simulink model "detectorDTMFv_nova"  (R2015a)
settings: Solver=ode45  StartTime=0.0  StopTime=10  RelTol=1e-3
undefined symbols (not defined in the file or in its folder): fa1
undefined symbols (not defined in the file): spf1
libraries: dsparch4 x12, dspvision x2, dspsrcs4 x2
settings Model: Creator=aluno  LastModifiedBy=aluno

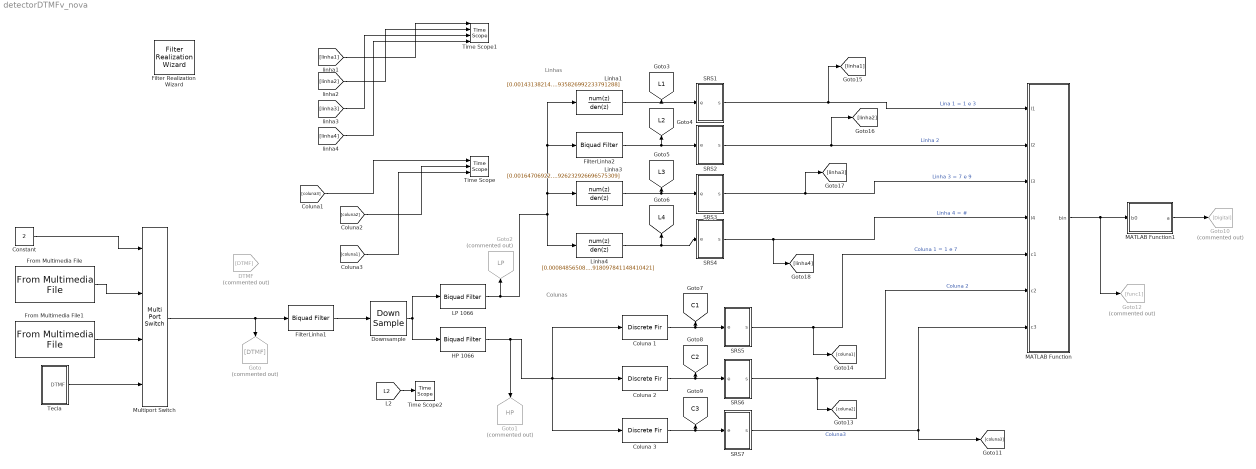
== system detectorDTMFv_nova ==
  note: Colunas
  note: Linhas
  Coluna 1 : DiscreteFir  Tag=BlockMethodSubSystem  Coefficients=[0.0162374776061879368 0.00189985661140890452 -0.00797907219847647162 -0.0052479937717645319 0.00711016072981206747 0.00994959173688526183 -0.004947856232688801 -0.0134569820625869124 -0.000253952320820913235 0.0161841189423569572 0.00648786614938951737 -0.015546033116355204 -0.0142422778845492579 0.0123011904003162455 0.020662915544833009 -0.00502839342402886316 -0.0254317147244396899 -0.00430154976592201765 0.0259053247088500034 0.0154089086154453655 -0.0223513453420253506 -0.0252581254312456739 0.0137329360710826773 0.0327518005541912877 -0.00195023169392464796 -0.0352357630400336602 -0.0120135916294035645 0.0324725455811842589 0.0250613597548236811 -0.0238106275094853714 -0.035341140965640179 0.0109201536347342254 0.0403511098959608225 0.00454288360450943313 -0.0393003808148319617 -0.0196726822859361571 0.0319801461843528603 0.0319801461843528603 -0.0196726822859361571 -0.0393003808148319617 0.00454288360450943313 0.0403511098959608225 0.0109201536347342254 -0.035341140965640179 -0.0238106275094853714 0.0250613597548236811 0.0324725455811842589 -0.0120135916294035645 -0.0352357630400336602 -0.00195023169392464796 0.0327518005541912877 0.0137329360710826773 -0.0252581254312456739 -0.0223513453420253506 0.0154089086154453655 0.0259053247088500034 -0.00430154976592201765 -0.0254317147244396899 -0.00502839342402886316 0.020662915544833009 0.0123011904003162455 -0.0142422778845492579 -0.015546033116355204 0.00648786614938951737 0.0161841189423569572 -0.000253952320820913235 -0.0134569820625869124 -0.004947856232688801 0.00994959173688526183 0.00711016072981206747 -0.0052479937717645319 -0.00797907219847647162 0.00189985661140890452 0.0162374776061879368]  InputProcessing=Columns as channels (frame based)
  Coluna 2 : DiscreteFir  Tag=BlockMethodSubSystem  Coefficients=[0.0151609358216046233 0.00947495343349298927 -0.0146508717306113884 -0.00105872890071495823 0.00918832200093996215 0.00869381341841268633 -0.0152655644424472808 -0.00814107176471721115 0.0147925932332998757 0.0127477000713067754 -0.0175823788993001162 -0.0151052177040993923 0.0180679752451277792 0.0192083709848808286 -0.0191711594948643961 -0.0227113888358491493 0.0191652238273957339 0.0267522427716407989 -0.0189311110191219371 -0.0305289457692412315 0.0179327879619009534 0.0342765820241483776 -0.0164300130975231704 -0.0376548966600824472 0.0143049369115090964 0.0406609187674431688 -0.0117262623087099286 -0.043127450615960447 0.00868997394253513689 0.0449559783178955022 -0.00535632534591356721 -0.046091514358570472 0.00181093739417893286 0.0464677162435992649 0.00181093739417893286 -0.046091514358570472 -0.00535632534591356721 0.0449559783178955022 0.00868997394253513689 -0.043127450615960447 -0.0117262623087099286 0.0406609187674431688 0.0143049369115090964 -0.0376548966600824472 -0.0164300130975231704 0.0342765820241483776 0.0179327879619009534 -0.0305289457692412315 -0.0189311110191219371 0.0267522427716407989 0.0191652238273957339 -0.0227113888358491493 -0.0191711594948643961 0.0192083709848808286 0.0180679752451277792 -0.0151052177040993923 -0.0175823788993001162 0.0127477000713067754 0.0147925932332998757 -0.00814107176471721115 -0.0152655644424472808 0.00869381341841268633 0.00918832200093996215 -0.00105872890071495823 -0.0146508717306113884 0.00947495343349298927 0.0151609358216046233]  InputProcessing=Columns as channels (frame based)
  Coluna 3 : DiscreteFir  Tag=BlockMethodSubSystem  Coefficients=[0.00988513023850831618 -0.0150839385628058591 -0.012276056219741845 0.00793493611486074772 0.00624928738101373886 -0.0154557718125388887 -0.00580602331170108898 0.0194847183612866931 0.00170258274655131253 -0.0239671147608122893 0.00374191930103570658 0.0270475037862077383 -0.0109223335109471052 -0.028320544283840763 0.0191883198599795482 0.0272259567957319551 -0.0278505151864056333 -0.0234560510640422493 0.0360331366276040732 0.0169923009575104825 -0.0428124432863375426 -0.0081801447891480146 0.0473482486516168463 -0.00236615855399630731 -0.0489985066204024072 0.0137299516321145107 0.0473977728496665293 -0.0248925638188108173 -0.0425415916558437579 0.0348110051185492875 0.0348110051185492875 -0.0425415916558437579 -0.0248925638188108173 0.0473977728496665293 0.0137299516321145107 -0.0489985066204024072 -0.00236615855399630731 0.0473482486516168463 -0.0081801447891480146 -0.0428124432863375426 0.0169923009575104825 0.0360331366276040732 -0.0234560510640422493 -0.0278505151864056333 0.0272259567957319551 0.0191883198599795482 -0.028320544283840763 -0.0109223335109471052 0.0270475037862077383 0.00374191930103570658 -0.0239671147608122893 0.00170258274655131253 0.0194847183612866931 -0.00580602331170108898 -0.0154557718125388887 0.00624928738101373886 0.00793493611486074772 -0.012276056219741845 -0.0150839385628058591 0.00988513023850831618]  InputProcessing=Columns as channels (frame based)
  Constant : Constant  Value=2
  DTMF : From  Commented=on  GotoTag=DTMF
  Downsample : DownSample  N=8  RateOptions=Allow multirate processing
  Filter Realization Wizard : dsparch4/Filter Realization Wizard
  FilterLinha1 : dsparch4/Biquad Filter  Tag=BlockMethodSubSystem  IIRFiltStruct=Direct form II  CoeffSource=Specify via dialog  BiQuadCoeffs=[1 2 1 1 -1.77399903150737015 0.912639318363765439;1 2 1 1 -1.76215470273778285 0.79641905117053291]  a0Flag=Warning  IC=0  ICnum=0  ICden=0  InputProcessing=Columns as channels (frame based)  denAccumFracLength=30  denProdOutputFracLength=30  secondMemoryFracLength=15  roundingMode=Floor  overflowMode=off  ScaleValues=[0.0346600717140988085;0.00856608710818747114;0.841395141645195133]  optimizeScaleValues=on  ScaleValueMode=Specify via input port (g)  scaleValueFracLength=14  FilterSource=Specify via dialog  FilterObject=Hm_biquad
  FilterLinha2 : dsparch4/Biquad Filter  Tag=BlockMethodSubSystem  IIRFiltStruct=Direct form II  CoeffSource=Specify via dialog  BiQuadCoeffs=[1 -1.4206643064571538 1 1 -1.25491628037472003 0.985502558796195638;1 -1.1033582980484935 1 1 -1.27745221072506698 0.985676226822505219]  a0Flag=Warning  IC=0  ICnum=0  ICden=0  InputProcessing=Columns as channels (frame based)  denAccumFracLength=30  denProdOutputFracLength=30  secondMemoryFracLength=15  roundingMode=Floor  overflowMode=off  ScaleValues=[0.0998036605233421636;0.0998036605233421636;1]  optimizeScaleValues=on  ScaleValueMode=Specify via input port (g)  scaleValueFracLength=14  FilterSource=Specify via dialog  FilterObject=Hm_biquad
  From Multimedia File : dspvision/From Multimedia File  inputFilename=/home/aluno/Downloads/DTMF.ogg  loop=on  numPlays=inf  outputStreams=Audio only  videoDataType=single  audioDataType=double  inheritSampleTime=on  userDefinedSampleTime=1/30  noAudioOutput=off  isIntensityVideo=off  fourcc=RGB  colorVideoFormat=Separate color signals  outputEOF=off  dataOrg=Column-major  audioFrameSize=spf1  computeAudioFrameSize=off  outSamplingMode=Sample based
  From Multimedia File1 : dspvision/From Multimedia File  inputFilename=/home/aluno/Downloads/7913#.ogg  loop=on  numPlays=inf  outputStreams=Audio only  videoDataType=single  audioDataType=double  inheritSampleTime=on  userDefinedSampleTime=1/30  noAudioOutput=off  isIntensityVideo=off  fourcc=RGB  colorVideoFormat=Separate color signals  outputEOF=off  dataOrg=Column-major  audioFrameSize=spf1  computeAudioFrameSize=off  outSamplingMode=Sample based
  Goto : Goto  Commented=on  GotoTag=DTMF
  Goto1 : Goto  Commented=on  GotoTag=HP  TagVisibility=global
  Goto10 : Goto  Commented=on  GotoTag=Digital
  Goto12 : Goto  Commented=on  GotoTag=func1
  Goto2 : Goto  Commented=on  GotoTag=LP  TagVisibility=global
  HP 1066 : dsparch4/Biquad Filter  Tag=BlockMethodSubSystem  IIRFiltStruct=Direct form II  CoeffSource=Specify via dialog  BiQuadCoeffs=[1 -2 1 1 -0.584098631504043841 0.792871341403187047;1 -2 1 1 0.426036160749820147 0.290070169958779767]  a0Flag=Warning  IC=0  ICnum=0  ICden=0  InputProcessing=Columns as channels (frame based)  denAccumFracLength=30  denProdOutputFracLength=30  secondMemoryFracLength=15  roundingMode=Floor  overflowMode=off  ScaleValues=[0.594242493226807778;0.216008502302239891;0.841395141645195133]  optimizeScaleValues=on  ScaleValueMode=Specify via input port (g)  scaleValueFracLength=14  FilterSource=Specify via dialog  FilterObject=Hm_biquad
  LP 1066 : dsparch4/Biquad Filter  Tag=BlockMethodSubSystem  IIRFiltStruct=Direct form II  CoeffSource=Specify via dialog  BiQuadCoeffs=[1 2 1 1 -0.665333766450005193 0.79613348517815774;1 2 1 1 -1.16290921522145752 0.47295210928305087]  a0Flag=Warning  IC=0  ICnum=0  ICden=0  InputProcessing=Columns as channels (frame based)  denAccumFracLength=30  denProdOutputFracLength=30  secondMemoryFracLength=15  roundingMode=Floor  overflowMode=off  ScaleValues=[0.282699929682038165;0.0775107235153982832;0.841395141645195133]  optimizeScaleValues=on  ScaleValueMode=Specify via input port (g)  scaleValueFracLength=14  FilterSource=Specify via dialog  FilterObject=Hm_biquad
  Linha1 : DiscreteFilter  Tag=BlockMethodSubSystem  Numerator=[0.00143138214148962246 -0.00399928386900759263 0.00421549467129527129 0 -0.00421549467129527129 0.00399928386900759263 -0.00143138214148962246]  Denominator=[1 -4.15803677575891317 8.69712495446401412 -10.7962985508542388 8.50695759347203584 -3.9781853030165335 0.935826992233791288]  InputProcessing=Columns as channels (frame based)  a0EqualsOne=on
  Linha3 : DiscreteFilter  Tag=BlockMethodSubSystem  Numerator=[0.00164706922346999091 -0.00370526492343735631 0.00371166563158928245 0 -0.00371166563158928245 0.00370526492343735631 -0.00164706922346999091]  Denominator=[1 -3.34565745513575852 6.65482815014997531 -7.90884772414054105 6.48700170175998547 -3.17902828471224197 0.926232926696575309]  InputProcessing=Columns as channels (frame based)  a0EqualsOne=on
  Linha4 : DiscreteFilter  Tag=BlockMethodSubSystem  Numerator=[0.000848565081379532146 -0.00160409606198937496 0.00157713327916364325 -6.54306174870359165e-21 -0.00157713327916364325 0.00160409606198937496 -0.000848565081379532146]  Denominator=[1 -2.82691943332089002 5.57865613790708803 -6.33091320195414919 5.42200709739372488 -2.67037232087107812 0.918097841148410421]  InputProcessing=Columns as channels (frame based)  a0EqualsOne=on
  MATLAB Function : MATLAB Function  TreatAsAtomicUnit=on
  MATLAB Function1 : MATLAB Function  TreatAsAtomicUnit=on
  Multiport Switch : MultiPortSwitch
  SRS1 : Subsystem
  SRS2 : Subsystem
  SRS3 : Subsystem
  SRS4 : Subsystem
  SRS5 : Subsystem
  SRS6 : Subsystem
  SRS7 : Subsystem
  Tecla : Subsystem  mask{linha=697, coluna=1209, spf1=spf1, fa1=fa1}
      mask prompts: linha "Frequencia da linha [linha]"; coluna "Frequencia da coluna [coluna]"; spf1 "Amostras por quadro [spf1]"; fa1 "Frequencia de Amostragem [fa1]"
  Time Scope : TimeScope  DefaultConfigurationName=spbscopes.TimeScopeBlockCfg  NumInputPorts=3
  Time Scope1 : TimeScope  DefaultConfigurationName=spbscopes.TimeScopeBlockCfg  NumInputPorts=4
  Time Scope2 : TimeScope  DefaultConfigurationName=spbscopes.TimeScopeBlockCfg
  tag scope: C1=global, C2=global, C3=global, L1=global, L2=global, L3=global, L4=global
  wires:
  Constant/1 -> Multiport Switch/1
  From Multimedia File/1 -> Multiport Switch/2
  From Multimedia File1/1 -> Multiport Switch/3
  Tecla/1(DTMF) -> Multiport Switch/4
  FilterLinha1/1 -> Downsample/1
  Multiport Switch/1 -> FilterLinha1/1, Goto/1
  Downsample/1 -> HP 1066/1, LP 1066/1
  SRS4/1(s) -> [linha4], MATLAB Function/4(l4)  "Linha 4 = #"
  SRS3/1(s) -> [linha3], MATLAB Function/3(l3)  "Linha 3 = 7 e 9"
  SRS2/1(s) -> [linha2], MATLAB Function/2(l2)  "Linha 2"
  SRS1/1(s) -> [linha1], MATLAB Function/1(l1)  "Lina 1 = 1 e 3"
  LP 1066/1 -> Goto2/1, Linha4/1, Linha3/1, FilterLinha2/1, Linha1/1
  SRS7/1(s) -> MATLAB Function/7(c3), [coluna3]  "Coluna3"
  SRS6/1(s) -> [coluna2], MATLAB Function/6(c2)  "Coluna 2"
  SRS5/1(s) -> [coluna1], MATLAB Function/5(c1)  "Coluna 1 = 1 e 7"
  Coluna 2/1 -> SRS6/1(e), [C2]
  Coluna 3/1 -> SRS7/1(e), [C3]
  Coluna 1/1 -> SRS5/1(e), [C1]
  HP 1066/1 -> Goto1/1, Coluna 3/1, Coluna 2/1, Coluna 1/1
  MATLAB Function/1(bin) -> Goto12/1, MATLAB Function1/1(b0)
  MATLAB Function1/1(a) -> Goto10/1
  Linha1/1 -> SRS1/1(e), [L1]
  Linha3/1 -> SRS3/1(e), [L3]
  Linha4/1 -> [L4], SRS4/1(e)
  [coluna3] -> Time Scope/1
  [coluna2] -> Time Scope/2
  [coluna1] -> Time Scope/3
  [linha1] -> Time Scope1/1
  [linha2] -> Time Scope1/2
  [linha3] -> Time Scope1/3
  [linha4] -> Time Scope1/4
  [L2] -> Time Scope2/1
  FilterLinha2/1 -> SRS2/1(e), [L2]

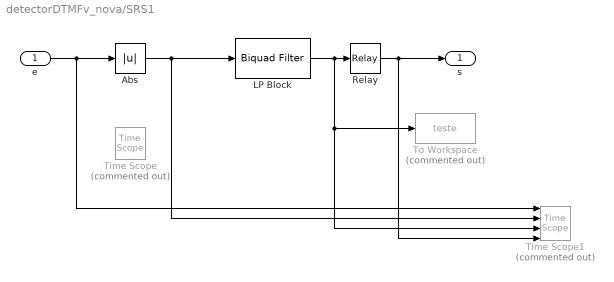
== system detectorDTMFv_nova/SRS1 ==
  e : Inport
  Abs : Abs
  LP Block : dsparch4/Biquad Filter  Tag=BlockMethodSubSystem  IIRFiltStruct=Direct form II  CoeffSource=Specify via dialog  BiQuadCoeffs=[1 2 1 1 -1.9659013837346071 0.967099117650403017]  a0Flag=Warning  IC=0  ICnum=0  ICden=0  InputProcessing=Columns as channels (frame based)  denAccumFracLength=30  denProdOutputFracLength=30  secondMemoryFracLength=15  roundingMode=Floor  overflowMode=off  ScaleValues=[0.000299433478949018132;0.841395141645195133]  optimizeScaleValues=on  ScaleValueMode=Specify via input port (g)  scaleValueFracLength=14  FilterSource=Specify via dialog  FilterObject=Hm_biquad
  Relay : Relay  OnSwitchValue=0.12  OffSwitchValue=0.05  ZeroCross=off
  Time Scope : TimeScope  Commented=on  DefaultConfigurationName=spbscopes.TimeScopeBlockCfg
  Time Scope1 : TimeScope  Commented=on  DefaultConfigurationName=spbscopes.TimeScopeBlockCfg  NumInputPorts=4
  To Workspace : ToWorkspace  Commented=on  VariableName=teste  SaveFormat=Timeseries  SampleTime=-1
  s : Outport
  wires:
  e/1 -> Time Scope1/1, Abs/1
  Abs/1 -> LP Block/1, Time Scope1/2
  Relay/1 -> Time Scope1/4, s/1
  LP Block/1 -> Relay/1, To Workspace/1, Time Scope1/3

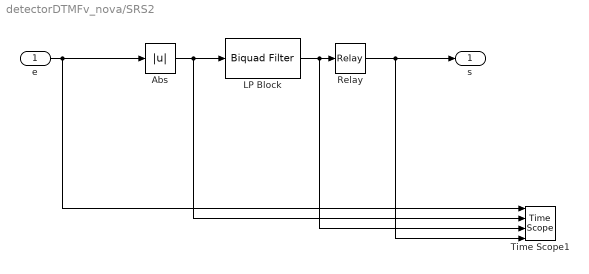
== system detectorDTMFv_nova/SRS2 ==
  e : Inport
  Abs : Abs
  LP Block : dsparch4/Biquad Filter  Tag=BlockMethodSubSystem  IIRFiltStruct=Direct form II  CoeffSource=Specify via dialog  BiQuadCoeffs=[1 2 1 1 -1.9659013837346071 0.967099117650403017]  a0Flag=Warning  IC=0  ICnum=0  ICden=0  InputProcessing=Columns as channels (frame based)  denAccumFracLength=30  denProdOutputFracLength=30  secondMemoryFracLength=15  roundingMode=Floor  overflowMode=off  ScaleValues=[0.000299433478949018132;0.841395141645195133]  optimizeScaleValues=on  ScaleValueMode=Specify via input port (g)  scaleValueFracLength=14  FilterSource=Specify via dialog  FilterObject=Hm_biquad
  Relay : Relay  OnSwitchValue=0.12  OffSwitchValue=0.05  ZeroCross=off
  Time Scope1 : TimeScope  DefaultConfigurationName=spbscopes.TimeScopeBlockCfg  NumInputPorts=4
  s : Outport
  wires:
  e/1 -> Time Scope1/1, Abs/1
  Abs/1 -> LP Block/1, Time Scope1/2
  Relay/1 -> Time Scope1/4, s/1
  LP Block/1 -> Time Scope1/3, Relay/1

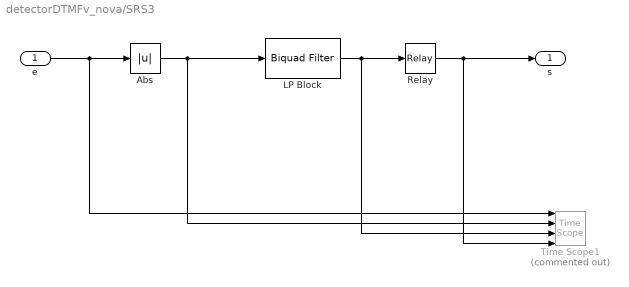
== system detectorDTMFv_nova/SRS3 ==
  e : Inport
  Abs : Abs
  LP Block : dsparch4/Biquad Filter  Tag=BlockMethodSubSystem  IIRFiltStruct=Direct form II  CoeffSource=Specify via dialog  BiQuadCoeffs=[1 2 1 1 -1.9659013837346071 0.967099117650403017]  a0Flag=Warning  IC=0  ICnum=0  ICden=0  InputProcessing=Columns as channels (frame based)  denAccumFracLength=30  denProdOutputFracLength=30  secondMemoryFracLength=15  roundingMode=Floor  overflowMode=off  ScaleValues=[0.000299433478949018132;0.841395141645195133]  optimizeScaleValues=on  ScaleValueMode=Specify via input port (g)  scaleValueFracLength=14  FilterSource=Specify via dialog  FilterObject=Hm_biquad
  Relay : Relay  OnSwitchValue=0.12  OffSwitchValue=0.05  ZeroCross=off
  Time Scope1 : TimeScope  Commented=on  DefaultConfigurationName=spbscopes.TimeScopeBlockCfg  NumInputPorts=4
  s : Outport
  wires:
  LP Block/1 -> Time Scope1/3, Relay/1
  e/1 -> Time Scope1/1, Abs/1
  Abs/1 -> LP Block/1, Time Scope1/2
  Relay/1 -> Time Scope1/4, s/1

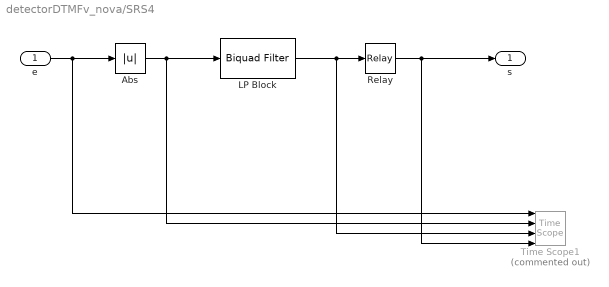
== system detectorDTMFv_nova/SRS4 ==
  e : Inport
  Abs : Abs
  LP Block : dsparch4/Biquad Filter  Tag=BlockMethodSubSystem  IIRFiltStruct=Direct form II  CoeffSource=Specify via dialog  BiQuadCoeffs=[1 2 1 1 -1.9659013837346071 0.967099117650403017]  a0Flag=Warning  IC=0  ICnum=0  ICden=0  InputProcessing=Columns as channels (frame based)  denAccumFracLength=30  denProdOutputFracLength=30  secondMemoryFracLength=15  roundingMode=Floor  overflowMode=off  ScaleValues=[0.000299433478949018132;0.841395141645195133]  optimizeScaleValues=on  ScaleValueMode=Specify via input port (g)  scaleValueFracLength=14  FilterSource=Specify via dialog  FilterObject=Hm_biquad
  Relay : Relay  OnSwitchValue=0.12  OffSwitchValue=0.05  ZeroCross=off
  Time Scope1 : TimeScope  Commented=on  DefaultConfigurationName=spbscopes.TimeScopeBlockCfg  NumInputPorts=4
  s : Outport
  wires:
  e/1 -> Time Scope1/1, Abs/1
  Abs/1 -> LP Block/1, Time Scope1/2
  Relay/1 -> Time Scope1/4, s/1
  LP Block/1 -> Time Scope1/3, Relay/1

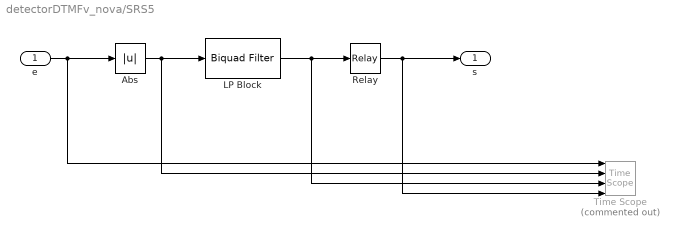
== system detectorDTMFv_nova/SRS5 ==
  e : Inport
  Abs : Abs
  LP Block : dsparch4/Biquad Filter  Tag=BlockMethodSubSystem  IIRFiltStruct=Direct form II  CoeffSource=Specify via dialog  BiQuadCoeffs=[1 2 1 1 -1.9659013837346071 0.967099117650403017]  a0Flag=Warning  IC=0  ICnum=0  ICden=0  InputProcessing=Columns as channels (frame based)  denAccumFracLength=30  denProdOutputFracLength=30  secondMemoryFracLength=15  roundingMode=Floor  overflowMode=off  ScaleValues=[0.000299433478949018132;0.841395141645195133]  optimizeScaleValues=on  ScaleValueMode=Specify via input port (g)  scaleValueFracLength=14  FilterSource=Specify via dialog  FilterObject=Hm_biquad
  Relay : Relay  OnSwitchValue=0.12  OffSwitchValue=0.05  ZeroCross=off
  Time Scope : TimeScope  Commented=on  DefaultConfigurationName=spbscopes.TimeScopeBlockCfg  NumInputPorts=4
  s : Outport
  wires:
  e/1 -> Time Scope/1, Abs/1
  Abs/1 -> LP Block/1, Time Scope/2
  Relay/1 -> Time Scope/4, s/1
  LP Block/1 -> Time Scope/3, Relay/1

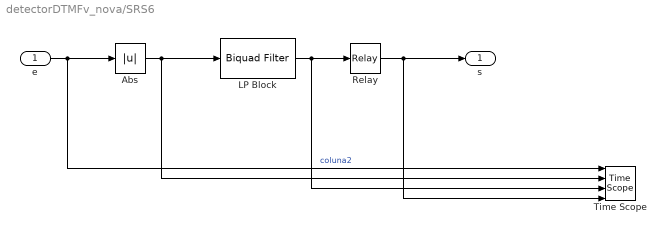
== system detectorDTMFv_nova/SRS6 ==
  e : Inport
  Abs : Abs
  LP Block : dsparch4/Biquad Filter  Tag=BlockMethodSubSystem  IIRFiltStruct=Direct form II  CoeffSource=Specify via dialog  BiQuadCoeffs=[1 2 1 1 -1.9659013837346071 0.967099117650403017]  a0Flag=Warning  IC=0  ICnum=0  ICden=0  InputProcessing=Columns as channels (frame based)  denAccumFracLength=30  denProdOutputFracLength=30  secondMemoryFracLength=15  roundingMode=Floor  overflowMode=off  ScaleValues=[0.000299433478949018132;0.841395141645195133]  optimizeScaleValues=on  ScaleValueMode=Specify via input port (g)  scaleValueFracLength=14  FilterSource=Specify via dialog  FilterObject=Hm_biquad
  Relay : Relay  OnSwitchValue=0.001  OffSwitchValue=0.0005  ZeroCross=off
  Time Scope : TimeScope  DefaultConfigurationName=spbscopes.TimeScopeBlockCfg  NumInputPorts=4
  s : Outport
  wires:
  e/1 -> Time Scope/1, Abs/1  "coluna2"
  Abs/1 -> LP Block/1, Time Scope/2
  Relay/1 -> Time Scope/4, s/1
  LP Block/1 -> Time Scope/3, Relay/1

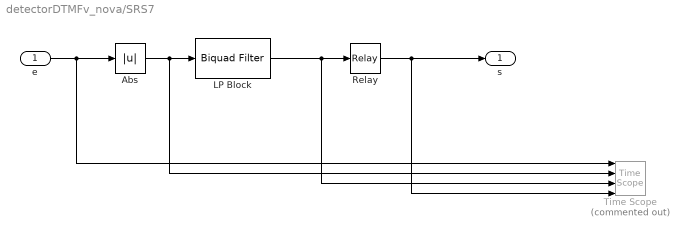
== system detectorDTMFv_nova/SRS7 ==
  e : Inport
  Abs : Abs
  LP Block : dsparch4/Biquad Filter  Tag=BlockMethodSubSystem  IIRFiltStruct=Direct form II  CoeffSource=Specify via dialog  BiQuadCoeffs=[1 2 1 1 -1.9659013837346071 0.967099117650403017]  a0Flag=Warning  IC=0  ICnum=0  ICden=0  InputProcessing=Columns as channels (frame based)  denAccumFracLength=30  denProdOutputFracLength=30  secondMemoryFracLength=15  roundingMode=Floor  overflowMode=off  ScaleValues=[0.000299433478949018132;0.841395141645195133]  optimizeScaleValues=on  ScaleValueMode=Specify via input port (g)  scaleValueFracLength=14  FilterSource=Specify via dialog  FilterObject=Hm_biquad
  Relay : Relay  OnSwitchValue=0.12  OffSwitchValue=0.05  ZeroCross=off
  Time Scope : TimeScope  Commented=on  DefaultConfigurationName=spbscopes.TimeScopeBlockCfg  NumInputPorts=4
  s : Outport
  wires:
  e/1 -> Time Scope/1, Abs/1
  Abs/1 -> LP Block/1, Time Scope/2
  Relay/1 -> Time Scope/4, s/1
  LP Block/1 -> Time Scope/3, Relay/1

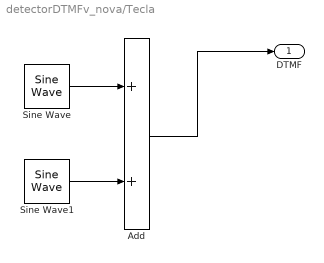
== system detectorDTMFv_nova/Tecla ==
  Add : Sum
  Sine Wave : dspsrcs4/Sine Wave  Amplitude=1  Frequency=coluna  Phase=0  SampleMode=Discrete  OutComplex=Real  CompMethod=Trigonometric fcn  TableSize=Speed  SampleTime=1/fa1  SamplesPerFrame=spf1  ResetState=Restart at time zero  dataType=double  wordLen=16  udDataType=sfix(16)  fracBitsMode=Best precision  numFracBits=15  OutDataTypeStr=double  LastOutDataTypeStr=double
  Sine Wave1 : dspsrcs4/Sine Wave  Amplitude=1  Frequency=linha  Phase=0  SampleMode=Discrete  OutComplex=Real  CompMethod=Trigonometric fcn  TableSize=Speed  SampleTime=1/fa1  SamplesPerFrame=spf1  ResetState=Restart at time zero  dataType=double  wordLen=16  udDataType=sfix(16)  fracBitsMode=Best precision  numFracBits=15  OutDataTypeStr=double  LastOutDataTypeStr=double
  DTMF : Outport
  wires:
  Sine Wave1/1 -> Add/2
  Sine Wave/1 -> Add/1
  Add/1 -> DTMF/1

== matlab function detectorDTMFv_nova/MATLAB Function1 ==
  data: b0 input; a output
function a = numero(b0)

a = bi2de(b0);
        
end

== matlab function detectorDTMFv_nova/MATLAB Function ==
  data: l1 input; bin output; l2 input; l3 input; l4 input; c1 input; c2 input; c3 input
function bin = digito(l1,l2,l3,l4,c1,c2,c3)

bin = zeros(size(l1,1),4);
for i = 1:size(l1,1)
decimal = bi2de([l1(i) l2(i) l3(i) l4(i) c1(i) c2(i) c3(i)]);
verifica = sum([l1(i) l2(i) l3(i) l4(i) c1(i) c2(i) c3(i)]);

switch (decimal)
    case 0 
        bin(1,:) = [0 0 0 0]; % 0   % nada foi selecionado
    case 17
        bin(i,:) = [1 0 0 0]; % 1   % linha 1 e coluna 1
    case 33
        bin(i,:) = [0 1 0 0]; % 2   % linha 1 e coluna 2
    case 65
        bin(i,:) = [1 1 0 0]; % 3   % linha 1 e coluna 3
    case 18
        bin(i,:) = [0 0 1 0]; % 4   % linha 2 e coluna 1
    case 34
        bin(i,:) = [1 0 1 0]; % 5   % linha 2 e coluna 2
    case 66
        bin(i,:) = [0 1 1 0]; % 6   % linha 2 e coluna 3
    case 20
        bin(i,:) = [1 1 1 0]; % 7   % linha 3 e coluna 1
    case 36
        bin(i,:) = [0 0 0 1]; % 8   % linha 3 e coluna 2
    case 68
        bin(i,:) = [1 0 0 1]; % 9   % linha 3 e coluna 3
    case 24 
        bin(i,:) = [0 1 0 1]; % 10  % linha 4 e coluna 2
    case 40
        bin(i,:) = [0 0 1 1]; %*    % linha 4 e coluna 1
    case 72
        bin(i,:) = [0 0 1 1]; % #   % linha 4 e coluna 3
   otherwise
        switch (verifica) % Erro
            case 1
                bin(i,:) = [1 0 1 1];
            case 2
                bin(i,:) = [1 1 1 1];
            otherwise
                bin(i,:) = [0 1 1 1];
        end
    end
end
